simulink model "Plant_angle"  (R2025b)
settings: Solver=FixedStepAuto  StartTime=0.0  StopTime=1000  FixedStep=simStepSize  RelTol=1e-3
undefined symbols (not defined in the file): initialAngle_deg, initialVehicleVelocity
libraries: autolibshared x1, dspstat3 x1
settings Model: DataDictionary=RL_data.sldd  Creator=Jacob  LastModifiedBy=scb548
settings RTWCC: GPUComputeCapability=3.5

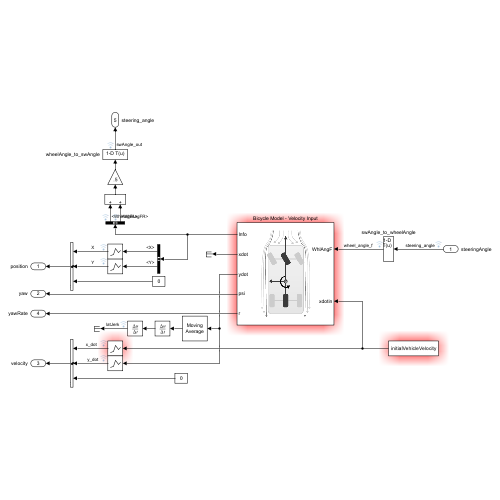
[thumbnail: Simulink's stored preview of the top-level diagram]
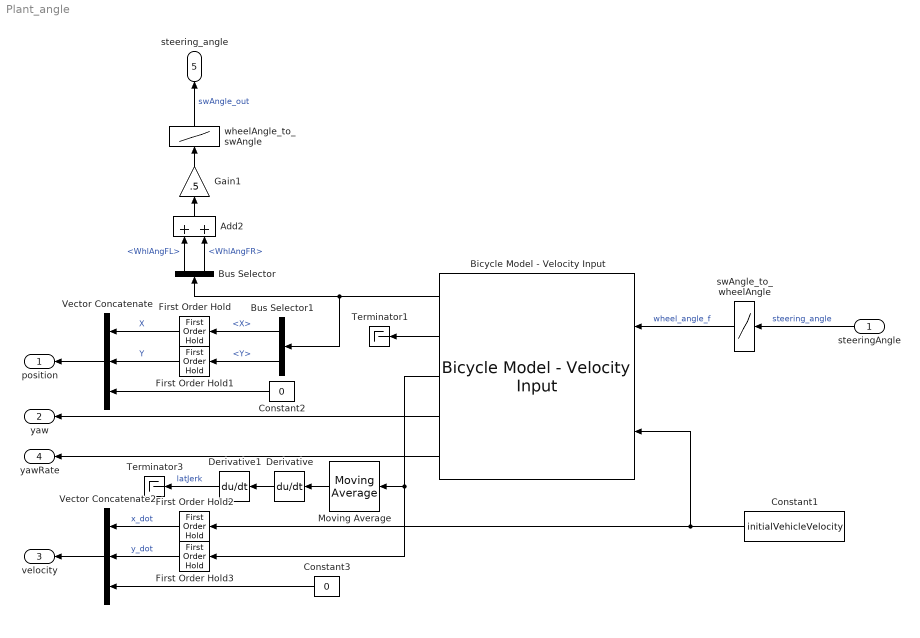
== system Plant_angle ==
  steeringAngle : Inport
  Add2 : Sum
  Bicycle Model - Velocity Input : autolibshared/Bicycle Model - Velocity Input  trackMode=Single (bicycle)  inputMode=External longitudinal velocity  frontSteerMode=on  rearSteerMode=off  windMode=off  muMode=off  extFMode=off  extMMode=off  aMode=3  NF=2  NR=2  m=2765.4  a=1.507  b=1.587  h=0.182  X_o=0  xdot_o=0  CalphaMode=off  sigmaMode=on  w=[1.4,1.4]  Cy_f=12e3  Cy_r=11e3  sigma_f=.1  sigma_r=.1  alpha_f_brk=[-.1 .1]  Cy_f_data=[-9e3 9e3]  alpha_r_brk=[-.1 .1]  Cy_r_data=[-9e3 9e3]  Y_o=0  ydot_o=0  Izz=4000  psi_o=initialAngle_deg*pi/180  r_o=0  Af=2  Cd=.3  Cl=.1  Cpm=.1  beta_w=[0 0.01:0.01:0.3]  Cs=[0 0.01:0.01:0.3]  Cym=[0 1e-6:0.01:0.3]  Pabs=101325  Tair=273  g=9.81  mu=1  xdot_tol=.01  Fznom=5000  Fxtire_sat=1e6  Fytire_sat=1e6  longOff=888.7  latOff=-143.6  vertOff=0
      settings: LibrarySourceBlock=drivingscenarioandsensors/Bicycle Model - Velocity Input
  Bus Selector : BusSelector  OutputSignals=BdyFrm.FrntAxl.Steer.WhlAngFL,BdyFrm.FrntAxl.Steer.WhlAngFR
  Bus Selector1 : BusSelector  OutputSignals=InertFrm.Cg.Disp.X,InertFrm.Cg.Disp.Y
  Constant1 : Constant  Value=initialVehicleVelocity
  Constant2 : Constant  Value=0
  Constant3 : Constant  Value=0
  Derivative : Derivative
  Derivative1 : Derivative
  First Order Hold : FirstOrderHold  ErrorTolerance=inf  AllowContinuousInput=on
  First Order Hold1 : FirstOrderHold  ErrorTolerance=inf  AllowContinuousInput=on
  First Order Hold2 : FirstOrderHold  InitialOutput=initialVehicleVelocity  ErrorTolerance=inf  AllowContinuousInput=on
  First Order Hold3 : FirstOrderHold  ErrorTolerance=inf  AllowContinuousInput=on
  Gain1 : Gain  Gain=.5
  Moving Average : dspstat3/Moving Average  Method=Sliding window  ForgettingFactorPort=off  SpecifyWindowLength=on  WindowLength=4  OverlapLength=3  AllowArbitraryInputLength=off  ForgettingFactor=0.9  SimulateUsing=Interpreted execution
  Terminator1 : Terminator
  Terminator3 : Terminator
  Vector Concatenate : Concatenate  NumInputs=3  Mode=Multidimensional array  ConcatenateDimension=2
  Vector Concatenate2 : Concatenate  NumInputs=3  Mode=Multidimensional array  ConcatenateDimension=2
  swAngle_to_wheelAngle : Lookup_n-D  NumberOfTableDimensions=1  BreakpointsForDimension1=[-10.89089966;-10.16600037;-9.441100121;-8.716199875;-7.991300106;-7.26639986;-6.541500092;-5.816599846;-5.091700077;-4.366799831;-3.641900063;-2.917000055;-2.192100048;-1.467200041;-0.742299974;-0.0175;0.0175;0.742299974;1.467200041;2.192100048;2.917000055;3.641900063;4.366799831;5.091700077;5.816599846;6.541500092;7.26639986;7.991300106;8.716199875;9.441100121;10.16600037;10.89089966]  Table=[-0.636900008;-0.589100003;-0.539099991;-0.490500003;-0.44659999;-0.404900014;-0.361499995;-0.317299992;-0.27610001;-0.237499997;-0.197899997;-0.156399995;-0.1162;-0.078699999;-0.041099999;-0.001;0.001;0.041200001;0.079099998;0.116499998;0.156399995;0.197999999;0.237900004;0.276499987;0.317400008;0.361499995;0.405299991;0.447100013;0.490700006;0.539099991;0.589399993;0.637499988]  InternalRulePriority=Speed  RndMeth=Simplest
  wheelAngle_to_swAngle : Lookup_n-D  NumberOfTableDimensions=1  BreakpointsForDimension1=[-0.636900008;-0.589100003;-0.539099991;-0.490500003;-0.44659999;-0.404900014;-0.361499995;-0.317299992;-0.27610001;-0.237499997;-0.197899997;-0.156399995;-0.1162;-0.078699999;-0.041099999;-0.001;0.001;0.041200001;0.079099998;0.116499998;0.156399995;0.197999999;0.237900004;0.276499987;0.317400008;0.361499995;0.405299991;0.447100013;0.490700006;0.539099991;0.589399993;0.637499988]  Table=[-10.89089966;-10.16600037;-9.441100121;-8.716199875;-7.991300106;-7.26639986;-6.541500092;-5.816599846;-5.091700077;-4.366799831;-3.641900063;-2.917000055;-2.192100048;-1.467200041;-0.742299974;-0.0175;0.0175;0.742299974;1.467200041;2.192100048;2.917000055;3.641900063;4.366799831;5.091700077;5.816599846;6.541500092;7.26639986;7.991300106;8.716199875;9.441100121;10.16600037;10.89089966]  InternalRulePriority=Speed  RndMeth=Simplest
  position : Outport
  yaw : Outport  Port=2
  velocity : Outport  Port=3
  yawRate : Outport  Port=4
  steering_angle : Outport  Port=5
  wires:
  Bus Selector/1 -> Add2/1  "<WhlAngFL>"
  First Order Hold1/1 -> Vector Concatenate/2  "Y"
  First Order Hold/1 -> Vector Concatenate/1  "X"
  Constant1/1 -> Bicycle Model - Velocity Input/2, First Order Hold2/1
  Bicycle Model - Velocity Input/1 -> Bus Selector/1, Bus Selector1/1
  Add2/1 -> Gain1/1
  Gain1/1 -> wheelAngle_to_swAngle/1
  Bus Selector1/2 -> First Order Hold1/1  "<Y>"
  Constant3/1 -> Vector Concatenate2/3
  Bus Selector1/1 -> First Order Hold/1  "<X>"
  Vector Concatenate2/1 -> velocity/1
  Constant2/1 -> Vector Concatenate/3
  Bicycle Model - Velocity Input/5 -> yawRate/1
  Vector Concatenate/1 -> position/1
  First Order Hold2/1 -> Vector Concatenate2/1  "x_dot"
  Bicycle Model - Velocity Input/4 -> yaw/1
  Bicycle Model - Velocity Input/3 -> Moving Average/1, First Order Hold3/1
  Bus Selector/2 -> Add2/2  "<WhlAngFR>"
  First Order Hold3/1 -> Vector Concatenate2/2  "y_dot"
  Bicycle Model - Velocity Input/2 -> Terminator1/1
  Derivative/1 -> Derivative1/1
  Derivative1/1 -> Terminator3/1  "latJerk"
  Moving Average/1 -> Derivative/1
  steeringAngle/1 -> swAngle_to_wheelAngle/1  "steering_angle"
  swAngle_to_wheelAngle/1 -> Bicycle Model - Velocity Input/1  "wheel_angle_f"
  wheelAngle_to_swAngle/1 -> steering_angle/1  "swAngle_out"
